simulink model "Ackeraman"  (R2019b)
settings: Solver=VariableStepAuto  StartTime=0.0  StopTime=simTime  RelTol=1e-3
values from neighbouring files (symbols this model uses):
  a0 = 1    [Ackerman_init.m]
  a1 = 4    [Ackerman_init.m]
  a2 = 3    [Ackerman_init.m]
  Change = 0    [Ackerman_init.m]
  k0 = 5    [Ackerman_init.m]
  k1 = place(Ad,bd,pd)    [Ackerman_init.m]
  k2 = place(Ac,bc,lambdatr')    [Ackerman_init.m]
  l = xlabel('Time (s)')    [Ackerman_init.m]
  pathType = 1    [Ackerman_init.m]
  phi0 = 0    [Ackerman_init.m]
  r = 2    [Ackerman_init.m]
  ref0 = [0 0]'    [Ackerman_init.m]
  refType = 1    [Ackerman_init.m]
  T = 0.3    [Ackerman_init.m]
  theta0 = pi    (= 3.14159265359)    [Ackerman_init.m]
  v0 = 2    [Ackerman_init.m]
  v_ref = 2    [Ackerman_init.m]
  x0 = 1    [Ackerman_init.m]
  y0 = 2    [Ackerman_init.m]
libraries: robotmobilelib x4
(part 1 of 4)
settings Model: Creator=mohd-  LastModifiedBy=mohd-

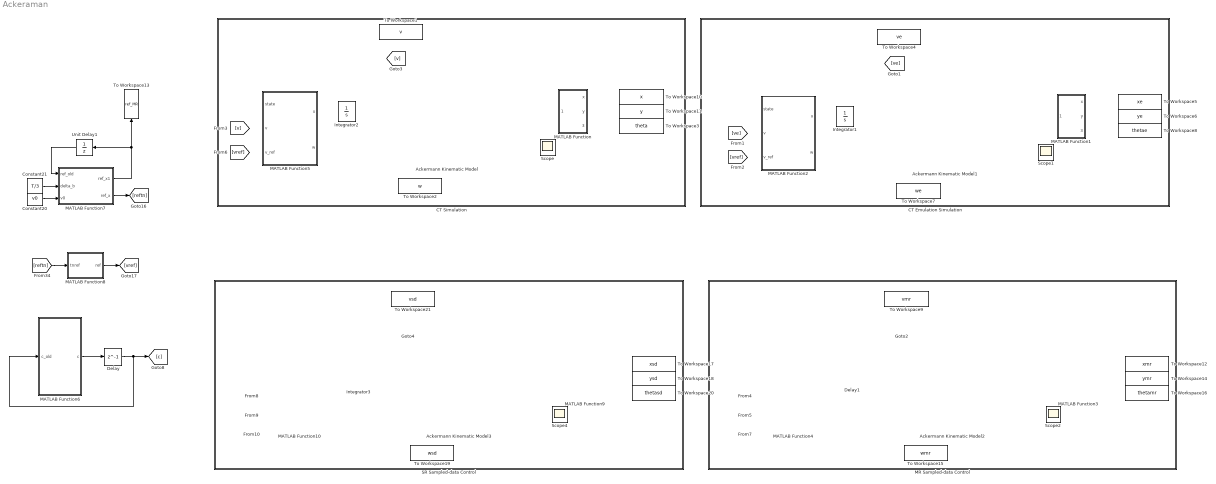
== system Ackeraman ==
  Ackermann Kinematic Model{,1..3} (4 alike) : robotmobilelib/Ackermann Kinematic Model  WheelBase=l  VehicleSpeedRange=[-inf inf]  MaxSteeringAngle=pi/3  InitialState=[x0; y0; theta0; phi0]  SimulateUsing=Interpreted execution
      settings: SourceProductName=Robotics System Toolbox  SourceProductBaseCode=RO
  CT Emulation Simulation : Subsystem
  CT Simulation : Subsystem
  Constant20 : Constant  Value=v0
  Constant21 : Constant  Value=T/3
  Delay : Delay  DelayLength=1  InitialCondition=0  SampleTime=T/3
  Delay1 : Delay  DelayLength=1  InitialCondition=v0  SampleTime=T
  Integrator1 : Integrator  InitialCondition=v0
  Integrator2 : Integrator  InitialCondition=v0
  Integrator3 : Integrator  InitialCondition=v0
  MATLAB Function : MATLAB Function  TreatAsAtomicUnit=on
  MATLAB Function1 : MATLAB Function  TreatAsAtomicUnit=on
  MATLAB Function10 : MATLAB Function  TreatAsAtomicUnit=on  SystemSampleTime=T
  MATLAB Function2 : MATLAB Function  TreatAsAtomicUnit=on  SystemSampleTime=T
  MATLAB Function3 : MATLAB Function  TreatAsAtomicUnit=on
  MATLAB Function4 : MATLAB Function  TreatAsAtomicUnit=on  SystemSampleTime=T
  MATLAB Function5 : MATLAB Function  TreatAsAtomicUnit=on
  MATLAB Function6 : MATLAB Function  TreatAsAtomicUnit=on  SystemSampleTime=T/3
  MATLAB Function7 : MATLAB Function  TreatAsAtomicUnit=on  SystemSampleTime=T
  MATLAB Function8 : MATLAB Function  TreatAsAtomicUnit=on
  MATLAB Function9 : MATLAB Function  TreatAsAtomicUnit=on
  MR Sampled-data Control : Subsystem
  SR Sampled-data Control : Subsystem
  Scope{,1..2,4} (4 alike) : Scope
  To Workspace1 : ToWorkspace  VariableName=v  SampleTime=10^-3
      settings: Save2DSignal=2-D array (concatenate along first dimension)
  To Workspace10 : ToWorkspace  VariableName=x  SampleTime=10^-3
      settings: Save2DSignal=2-D array (concatenate along first dimension)
  To Workspace11 : ToWorkspace  VariableName=y  SampleTime=10^-3
      settings: Save2DSignal=2-D array (concatenate along first dimension)
  To Workspace12 : ToWorkspace  VariableName=xmr  SampleTime=10^-3
      settings: Save2DSignal=2-D array (concatenate along first dimension)
  To Workspace13 : ToWorkspace  VariableName=ref_MR  SampleTime=T/3
  To Workspace14 : ToWorkspace  VariableName=ymr  SampleTime=10^-3
      settings: Save2DSignal=2-D array (concatenate along first dimension)
  To Workspace15 : ToWorkspace  VariableName=wmr  SampleTime=10^-3
      settings: Save2DSignal=2-D array (concatenate along first dimension)
  To Workspace16 : ToWorkspace  VariableName=thetamr  SampleTime=10^-3
      settings: Save2DSignal=2-D array (concatenate along first dimension)
  To Workspace17 : ToWorkspace  VariableName=xsd  SampleTime=10^-3
      settings: Save2DSignal=2-D array (concatenate along first dimension)
  To Workspace18 : ToWorkspace  VariableName=ysd  SampleTime=10^-3
      settings: Save2DSignal=2-D array (concatenate along first dimension)
  To Workspace19 : ToWorkspace  VariableName=wsd  SampleTime=10^-3
      settings: Save2DSignal=2-D array (concatenate along first dimension)
  To Workspace2 : ToWorkspace  VariableName=w  SampleTime=10^-3
      settings: Save2DSignal=2-D array (concatenate along first dimension)
  To Workspace20 : ToWorkspace  VariableName=thetasd  SampleTime=10^-3
      settings: Save2DSignal=2-D array (concatenate along first dimension)
  To Workspace21 : ToWorkspace  VariableName=vsd  SampleTime=10^-3
      settings: Save2DSignal=2-D array (concatenate along first dimension)
  To Workspace3 : ToWorkspace  VariableName=theta  SampleTime=10^-3
      settings: Save2DSignal=2-D array (concatenate along first dimension)
  To Workspace4 : ToWorkspace  VariableName=ve  SampleTime=10^-3
      settings: Save2DSignal=2-D array (concatenate along first dimension)
  To Workspace5 : ToWorkspace  VariableName=xe  SampleTime=10^-3
      settings: Save2DSignal=2-D array (concatenate along first dimension)
  To Workspace6 : ToWorkspace  VariableName=ye  SampleTime=10^-3
      settings: Save2DSignal=2-D array (concatenate along first dimension)
  To Workspace7 : ToWorkspace  VariableName=we  SampleTime=10^-3
      settings: Save2DSignal=2-D array (concatenate along first dimension)
  To Workspace8 : ToWorkspace  VariableName=thetae  SampleTime=10^-3
      settings: Save2DSignal=2-D array (concatenate along first dimension)
  To Workspace9 : ToWorkspace  VariableName=vmr  SampleTime=10^-3
      settings: Save2DSignal=2-D array (concatenate along first dimension)
  Unit Delay1 : UnitDelay  InitialCondition=ref0  SampleTime=T/3  HasFrameUpgradeWarning=on
  wires:
  Constant20/1 -> MATLAB Function7/3(v0)
  MATLAB Function8/1(ref) -> [vref]
  Constant21/1 -> MATLAB Function7/2(delta_b)
  Unit Delay1/1 -> MATLAB Function7/1(ref_old)
  MATLAB Function7/1(ref_x1) -> To Workspace13/1, Unit Delay1/1
  [reftn] -> MATLAB Function8/1(tnref)
  MATLAB Function7/2(ref_x) -> [reftn]
  MATLAB Function5/1(u) -> Integrator2/1
  MATLAB Function5/2(w) -> To Workspace2/1, Ackermann Kinematic Model/2
  Ackermann Kinematic Model/1 -> MATLAB Function5/1(state), MATLAB Function/1(state)
  Ackermann Kinematic Model/2 -> Scope/1
  Integrator2/1 -> To Workspace1/1, [v], Ackermann Kinematic Model/1
  [v] -> MATLAB Function5/2(v)
  [vref] -> MATLAB Function5/3(v_ref)
  MATLAB Function/2(y) -> To Workspace11/1
  MATLAB Function/1(x) -> To Workspace10/1
  MATLAB Function/3(theta) -> To Workspace3/1
  MATLAB Function2/2(w) -> To Workspace7/1, Ackermann Kinematic Model1/2
  [vref] -> MATLAB Function2/3(v_ref)
  [ve] -> MATLAB Function2/2(v)
  MATLAB Function2/1(u) -> Integrator1/1
  MATLAB Function1/3(theta) -> To Workspace8/1
  MATLAB Function1/1(x) -> To Workspace5/1
  Integrator1/1 -> To Workspace4/1, [ve], Ackermann Kinematic Model1/1
  Ackermann Kinematic Model1/2 -> Scope1/1
  MATLAB Function1/2(y) -> To Workspace6/1
  Ackermann Kinematic Model1/1 -> MATLAB Function2/1(state), MATLAB Function1/1(state)
  MATLAB Function3/2(y) -> To Workspace14/1
  Ackermann Kinematic Model2/1 -> MATLAB Function4/1(state), MATLAB Function3/1(state)
  Ackermann Kinematic Model2/2 -> Scope2/1
  MATLAB Function3/1(x) -> To Workspace12/1
  MATLAB Function4/1(u) -> Delay1/1
  [vmr] -> MATLAB Function4/2(v)
  Delay1/1 -> To Workspace9/1, [vmr], Ackermann Kinematic Model2/1
  MATLAB Function3/3(theta) -> To Workspace16/1
  [vref] -> MATLAB Function4/3(v_ref)
  MATLAB Function4/2(w) -> To Workspace15/1, Ackermann Kinematic Model2/2
  Delay/1 -> [c], MATLAB Function6/1(c_old)
  MATLAB Function6/1(c) -> Delay/1
  [c] -> MATLAB Function4/4(c)
  [c] -> MATLAB Function10/4(c)
  Ackermann Kinematic Model3/1 -> MATLAB Function10/1(state), MATLAB Function9/1(state)
  Integrator3/1 -> To Workspace21/1, [vsd], Ackermann Kinematic Model3/1
  MATLAB Function9/2(y) -> To Workspace18/1
  MATLAB Function9/3(theta) -> To Workspace20/1
  MATLAB Function10/2(w) -> To Workspace19/1, Ackermann Kinematic Model3/2
  [vref] -> MATLAB Function10/3(v_ref)
  MATLAB Function10/1(u) -> Integrator3/1
  [vsd] -> MATLAB Function10/2(v)
  MATLAB Function9/1(x) -> To Workspace17/1
  Ackermann Kinematic Model3/2 -> Scope4/1

== system Ackeraman/CT Emulation Simulation ==

== system Ackeraman/CT Simulation ==

== system Ackeraman/MR Sampled-data Control ==

== system Ackeraman/SR Sampled-data Control ==

== matlab function Ackeraman/MATLAB Function ==
  data: x output; state input; y output; theta output
function [x, y, theta] = fcn(state)

x = state(1);
y = state(2);
theta = state(3);

== matlab function Ackeraman/MATLAB Function5 ==
  data: state input; v input; v_ref input; pathType parameter; k0 parameter; a0 parameter; a1 parameter; a2 parameter; r parameter; l parameter; u output; w output; Change parameter; k2 parameter
function [u,w] = MATLAB_Function5(state, v, v_ref, pathType, k0, a0, a1, a2, r, l, Change, k2)

x = state(1); y = state(2); theta = state(3); phi = state(4);
eta1 = v;
if pathType == 1
    alpha = x^2+y^2 - r^2;
    dalpha = 2*v*(x*cos(theta) + y*sin(theta));
    ddalpha = (2*v^2*(l*cos(phi) + y*cos(theta)*sin(phi) - x*sin(phi)*sin(theta)))/(l*cos(phi));
    Lg1lfh2 = (2*eta1^2*(y*cos(theta) - x*sin(theta)))/(l*cos(phi)^2);
    Lf3     = -(2*eta1^3*sin(phi)^2*(x*cos(theta) + y*sin(theta)))/(l^2*cos(phi)^2);
else
    a       = 3; b       = 1.05*a;
    alpha = (x^2+y^2+a^2)^2-4*a^2*x^2-b^4; % defines the path
    dalpha = 4*v*y*sin(theta)*(a^2 + x^2 + y^2) + 4*v*x*cos(theta)*(- a^2 + x^2 + y^2);
    ddalpha = v*cos(theta)*(8*v*x^2*cos(theta) + 4*v*cos(theta)*(- a^2 + x^2 + y^2) + 8*v*x*y*sin(theta)) + v*sin(theta)*(4*v*sin(theta)*(a^2 + x^2 + y^2) + 8*v*y^2*sin(theta) + 8*v*x*y*cos(theta)) - (v*tan(phi)*(4*v*x*sin(theta)*(- a^2 + x^2 + y^2) - 4*v*y*cos(theta)*(a^2 + x^2 + y^2)))/l;
    Lg1lfh2 =  -(eta1*(tan(phi)^2 + 1)*(4*eta1*x*sin(theta)*(- a^2 + x^2 + y^2) - 4*eta1*y*cos(theta)*(a^2 + x^2 + y^2)))/l;
    Lf3     = -(4*eta1^3*(x^3*cos(theta)*sin(phi)^2 + y^3*sin(phi)^2*sin(theta) - 6*l^2*y*cos(phi)^2*sin(theta)^3 - 6*l^2*x*cos(phi)^2*cos(theta) - a^2*x*cos(theta)*sin(phi)^2 + a^2*y*sin(phi)^2*sin(theta) + x*y^2*cos(theta)*sin(phi)^2 + x^2*y*sin(phi)^2*sin(theta) - 6*l^2*y*cos(phi)^2*cos(theta)^2*sin(theta) - 6*a^2*l*cos(phi)*cos(theta)*sin(phi)*sin(theta) + 6*l*x^2*cos(phi)*cos(theta)*sin(phi)*sin(theta) - 6*l*y^2*cos(phi)*cos(theta)*sin(phi)*sin(theta) - 6*l*x*y*cos(phi)*cos(theta)^2*sin(phi) + 6*l*x*y*cos(phi)*sin(phi)*sin(theta)^2))/(l^2*cos(phi)^2);

end
if alpha < 1e-2 && Change == 1
    ref = 2*v_ref;
else
    ref = v_ref;
end

h = [alpha;dalpha;ddalpha];
u = -k0*(v-ref); 
v2 = k2*h;
w = (Lg1lfh2)^(-1)*(-Lf3+v2);

== matlab function Ackeraman/MATLAB Function1 ==
  data: x output; state input; y output; theta output
function [x, y, theta] = fcn(state)

x = state(1);
y = state(2);
theta = state(3);

== matlab function Ackeraman/MATLAB Function2 ==
  data: state input; v input; v_ref input; pathType parameter; k0 parameter; a0 parameter; a1 parameter; a2 parameter; r parameter; l parameter; u output; w output; Change parameter; k2 parameter
function [u,w] = MATLAB_Function5(state, v, v_ref, pathType, k0, a0, a1, a2, r, l, Change, k2)

x = state(1); y = state(2); theta = state(3); phi = state(4);
eta1 = v;
if pathType == 1
    alpha = x^2+y^2 - r^2;
    dalpha = 2*v*(x*cos(theta) + y*sin(theta));
    ddalpha = (2*v^2*(l*cos(phi) + y*cos(theta)*sin(phi) - x*sin(phi)*sin(theta)))/(l*cos(phi));
    Lg1lfh2 = (2*eta1^2*(y*cos(theta) - x*sin(theta)))/(l*cos(phi)^2);
    Lf3     = -(2*eta1^3*sin(phi)^2*(x*cos(theta) + y*sin(theta)))/(l^2*cos(phi)^2);
else
    a       = 3; b       = 1.05*a;
    alpha = (x^2+y^2+a^2)^2-4*a^2*x^2-b^4; % defines the path
    dalpha = 4*v*y*sin(theta)*(a^2 + x^2 + y^2) + 4*v*x*cos(theta)*(- a^2 + x^2 + y^2);
    ddalpha = v*cos(theta)*(8*v*x^2*cos(theta) + 4*v*cos(theta)*(- a^2 + x^2 + y^2) + 8*v*x*y*sin(theta)) + v*sin(theta)*(4*v*sin(theta)*(a^2 + x^2 + y^2) + 8*v*y^2*sin(theta) + 8*v*x*y*cos(theta)) - (v*tan(phi)*(4*v*x*sin(theta)*(- a^2 + x^2 + y^2) - 4*v*y*cos(theta)*(a^2 + x^2 + y^2)))/l;
    Lg1lfh2 =  -(eta1*(tan(phi)^2 + 1)*(4*eta1*x*sin(theta)*(- a^2 + x^2 + y^2) - 4*eta1*y*cos(theta)*(a^2 + x^2 + y^2)))/l;
    Lf3     = -(4*eta1^3*(x^3*cos(theta)*sin(phi)^2 + y^3*sin(phi)^2*sin(theta) - 6*l^2*y*cos(phi)^2*sin(theta)^3 - 6*l^2*x*cos(phi)^2*cos(theta) - a^2*x*cos(theta)*sin(phi)^2 + a^2*y*sin(phi)^2*sin(theta) + x*y^2*cos(theta)*sin(phi)^2 + x^2*y*sin(phi)^2*sin(theta) - 6*l^2*y*cos(phi)^2*cos(theta)^2*sin(theta) - 6*a^2*l*cos(phi)*cos(theta)*sin(phi)*sin(theta) + 6*l*x^2*cos(phi)*cos(theta)*sin(phi)*sin(theta) - 6*l*y^2*cos(phi)*cos(theta)*sin(phi)*sin(theta) - 6*l*x*y*cos(phi)*cos(theta)^2*sin(phi) + 6*l*x*y*cos(phi)*sin(phi)*sin(theta)^2))/(l^2*cos(phi)^2);

end
if alpha < 1e-2 && Change == 1
    ref = 2*v_ref;
else
    ref = v_ref;
end
h = [alpha;dalpha;ddalpha];
u = -k0*(v-ref); 
v2 = k2*h;
w = (Lg1lfh2)^(-1)*(-Lf3+v2);

== matlab function Ackeraman/MATLAB Function3 ==
  data: x output; state input; y output; theta output
function [x, y, theta] = fcn(state)

x = state(1);
y = state(2);
theta = state(3);
